simulink model "Two_ASK"  (R2013a)
settings: Solver=ode45  StartTime=0.0  StopTime=10.0  RelTol=1e-3
libraries: dsparch4 x1, commrandsrc2 x1, commsrccod2 x1
settings Model: Creator=sliencer  LastModifiedBy=sliencer

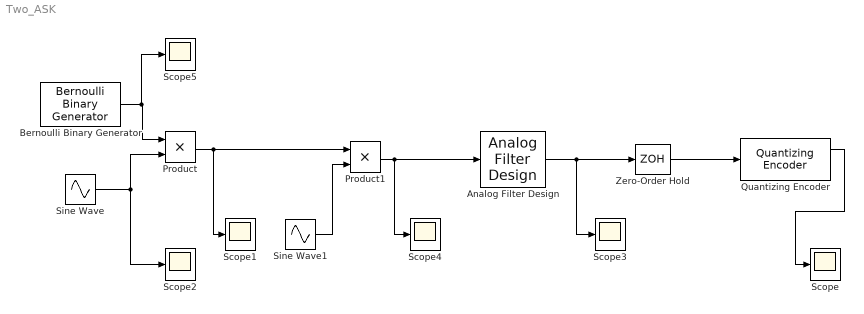
== system Two_ASK ==
  Analog Filter Design : dsparch4/Analog Filter Design  method=Butterworth  filttype=Lowpass  N=2  Wlo=30  Whi=80  Rp=2  Rs=40
  Bernoulli Binary Generator : commrandsrc2/Bernoulli Binary Generator  P=0.5  seed=61  Ts=1  frameBased=off  sampPerFrame=1  orient=off  outDataType=double
  Product : Product
  Product1 : Product
  Quantizing Encoder : commsrccod2/Quantizing Encoder  partition=[1]  codebook=[0 1]  idxDType=double
  Scope{,1..5} (6 alike) : Scope
      Scope2 settings: SaveName=ScopeData2
      Scope3 settings: SaveName=ScopeData3
      Scope4 settings: SaveName=ScopeData4
      Scope5 settings: SaveName=ScopeData5
  Sine Wave : Sin  Amplitude=2  Frequency=8*pi  SampleTime=1/500
  Sine Wave1 : Sin  Amplitude=2  Frequency=8*pi  SampleTime=1/500
  Zero-Order Hold : ZeroOrderHold
  wires:
  Bernoulli Binary Generator/1 -> Scope5/1, Product/1
  Sine Wave/1 -> Product/2, Scope2/1
  Product/1 -> Scope1/1, Product1/1
  Sine Wave1/1 -> Product1/2
  Product1/1 -> Scope4/1, Analog Filter Design/1
  Analog Filter Design/1 -> Scope3/1, Zero-Order Hold/1
  Zero-Order Hold/1 -> Quantizing Encoder/1
  Quantizing Encoder/1 -> Scope/1
